simulink model "LAFES"  (R2024a)
settings: Solver=FixedStepAuto  StartTime=0.0  StopTime=3600  FixedStep=0.01  RelTol=1e-3
PreLoadFcn:
  | addpath(genpath('./S_Functions'))
InitFcn:
  | NETIF =  'eth0';
model workspace (MAT data in the model file):
  Sig = Simulink.Signal
  Sig.DataType = 'auto'
  Sig.Dimensions = -1
  Sig.DimensionsMode = 'auto'
  Sig.Complexity = 'auto'
  Sig.SampleTime = -1
  Sig.SamplingMode = 'auto'
  link_id = 1
  main_switch = Simulink.Parameter
  main_switch.Value = 1
  main_switch.Complexity = 'real'
  main_switch.Dimensions = [1 1]
  main_switch.DataType = 'boolean'
  motor_e_stop = Simulink.Parameter
  motor_e_stop.Value = 0
  motor_e_stop.Complexity = 'real'
  motor_e_stop.Dimensions = [1 1]
  motor_e_stop.DataType = 'boolean'
  quick_stop = Simulink.Parameter
  quick_stop.Value = 0
  quick_stop.Complexity = 'real'
  quick_stop.Dimensions = [1 1]
  quick_stop.DataType = 'boolean'
  useGenerator = Simulink.Parameter
  useGenerator.Value = 1
  useGenerator.Complexity = 'real'
  useGenerator.Dimensions = [1 1]
  useGenerator.DataType = 'boolean'
settings Model: SimulationMode=external  Creator=20192648  LastModifiedBy=root
settings HardwareCC: ProdBitPerLong=64  ProdHWDeviceType=Intel->x86-64 (Linux 64)
settings ModelReferenceCC: EnableRefExpFcnMdlSchedulingChecks=on  PropagateSignalLabelsOutOfModel=off
settings RTWCC: Description=RoboCup Realtime Target  SystemTargetFile=mttarget.tlc  MakeCommand="make_rtw CC=\"ccache gcc\" OPTS=\"-DNETIF_ID=0 -DTEST_CONN_MODEL -D_GNU_SOURCE -DPRIO=99\""  TemplateMakefile=mt_unix.tmf  CustomInclude=./S_Functions  RTWCompilerOptimization=Custom  RTWCustomCompilerOptimizations=-O2 -g -W
settings RTWCC: CustomSource=|
  | Rs485EthercatLibrary.c
  | ethercatbase.c
  | ethercatcoe.c
  | ethercatconfig.c
  | ethercatdc.c
  | ethercatfoe.c
  | ethercatmain.c
  | ethercatprint.c
  | ethercatsoe.c
  | nicdrv.c
  | osal.c
  | oshw.c
  | timer_posix.c
  | timer_stats.c
settings CodeAppCC: StateflowObjectComments=on
settings GRTTargetCC: TargetLangStandard=C89/C90 (ANSI)  CodeReplacementLibrary=GNU C99 extensions  UseToolchainInfoCompliant=off  ExtMode=on

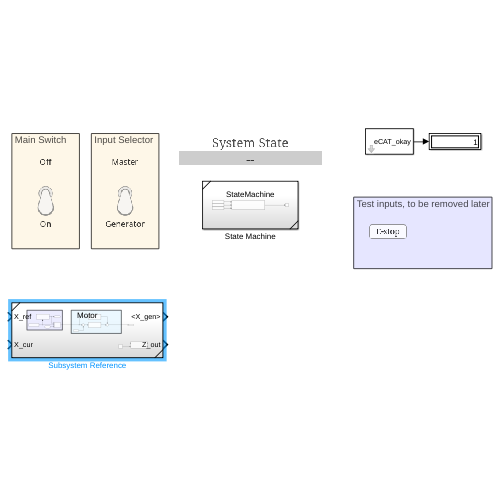
[thumbnail: Simulink's stored preview of the top-level diagram]
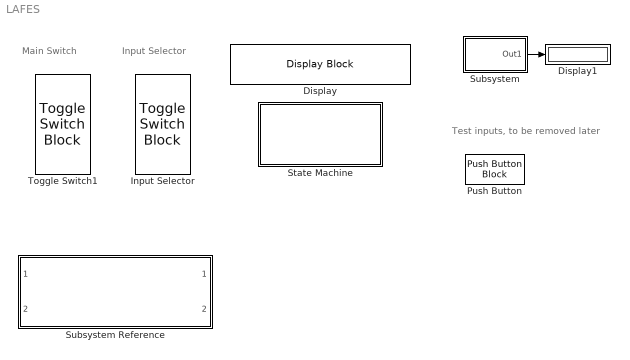
== system LAFES ==
  note: Test inputs, to be removed later
  note: Input Selector
  note: Main Switch
  Display : DisplayBlock  Transparency=1
  Display1 : Display
  Input Selector : ToggleSwitchBlock  LabelPosition=Hide
      settings: Values={{'Generator', 'Master'}, [1 0]}
  Push Button : PushButtonBlock  ButtonText=E-stop  OffValue=0.000000
  State Machine : Subsystem  ReferencedSubsystem=StateMachine
  Subsystem : Subsystem  mask{NETIF=NETIF}
  Subsystem Reference : Subsystem  ReferencedSubsystem=Motor
  Toggle Switch1 : ToggleSwitchBlock  LabelPosition=Hide
      settings: Values={{'On', 'Off'}, [1 0]}
  wires:
  Subsystem/1(Out1) -> Display1/1

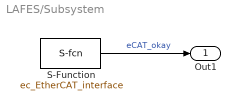
== system LAFES/Subsystem ==
  S-Function : S-Function  FunctionName=ec_EtherCAT_interface  Parameters=NETIF  SFunctionDeploymentMode=off  EnableBusSupport=off
  Out1 : Outport
  wires:
  S-Function/1 -> Out1/1  "eCAT_okay"
